simulink model "udp_test"  (R2022b)
settings: Solver=FixedStepAuto  StartTime=0.0  StopTime=100  FixedStep=Ts  RelTol=1e-3
InitFcn:
  | Ts = 1e-5;
  | Tc = 0.01;
undefined symbols (not defined in the file): f
libraries: slrealtimeutilitieslib x3, slrealtimeiplib x2, instrumentlib x1
settings Model: Creator=Javnson  LastModifiedBy=Javnson

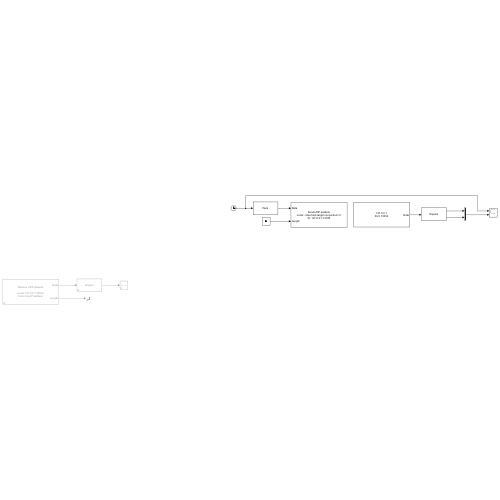
[thumbnail: Simulink's stored preview of the top-level diagram]
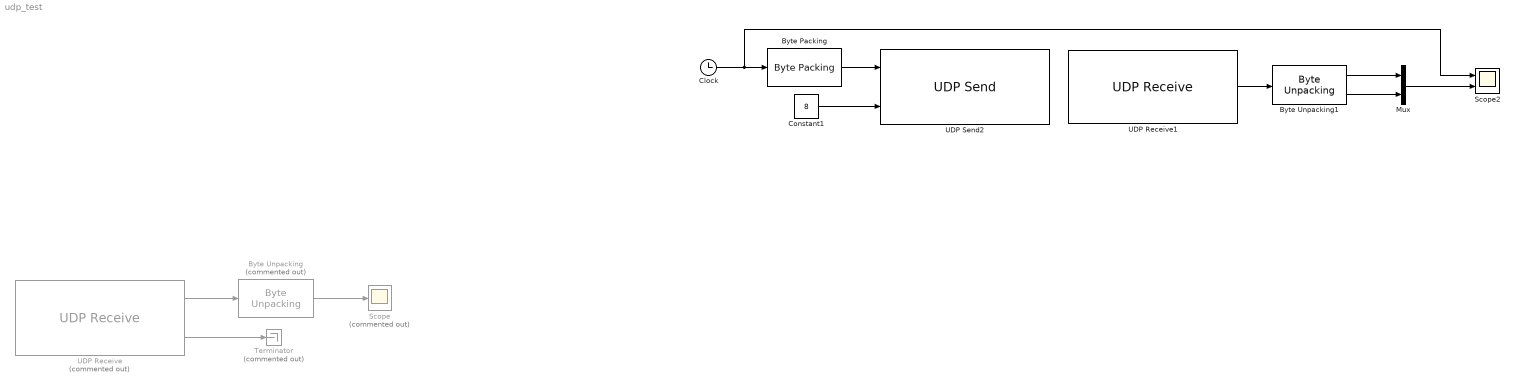
== system udp_test ==
  Byte Packing : slrealtimeutilitieslib/Byte Packing  MaskPackedDataType=uint8  MaskUnpackedDataTypes={'double'}  MaskAlignment=1
  Byte Unpacking : slrealtimeutilitieslib/Byte Unpacking  Commented=on  MaskUnpackedDataTypes={'double'}  MaskUnpackedDataSizes={[1]}  MaskAlignment=1
  Byte Unpacking1 : slrealtimeutilitieslib/Byte Unpacking  MaskUnpackedDataTypes={'double','double'}  MaskUnpackedDataSizes={[1],[1]}  MaskAlignment=1
  Clock : Clock
  Constant1 : Constant  Value=8
  Mux : Mux  Inputs=2
  Scope : Scope  Commented=on
  Scope2 : Scope  NumInputPorts=2
  Terminator : Terminator  Commented=on
  UDP Receive : slrealtimeiplib/UDP Receive  Commented=on  useHostTargetConn=off  ipAddress=127.0.0.1  localPort=10034  rcvWidth=8  rcvFmAny=on  fmAddress='10.10.10.10'  sampleTime=-1  enableMessage=off  maxPackets=1
  UDP Receive1 : instrumentlib/UDP Receive  LocalAddress=127.0.0.1  LocalPort=10034  EnablePortSharing=off  Host=localhost  Port=10034  GetLatestData=on  DataSize=[ 16 ]  DataType=int8  ASCIIFormatting=%f,  Terminator=LF  CustomTerminator=10  ByteOrder=little-endian  EnableBlockingMode=on  Timeout=100  SampleTime=Tc  SimulateUsing=Interpreted execution
  UDP Send2 : slrealtimeiplib/UDP Send  useHostTargetConn=on  toAddress='127.0.0.1'  toPort=10035  sampleTime=Tc  enableMessage=off
  wires:
  Byte Unpacking/1 -> Scope/1
  UDP Receive/2 -> Terminator/1
  UDP Receive/1 -> Byte Unpacking/1
  Clock/1 -> Scope2/1, Byte Packing/1
  Byte Packing/1 -> UDP Send2/1
  Constant1/1 -> UDP Send2/2
  UDP Receive1/1 -> Byte Unpacking1/1
  Byte Unpacking1/2 -> Mux/2
  Mux/1 -> Scope2/2
  Byte Unpacking1/1 -> Mux/1
